simulink model "motor_speed_current_loop_model"  (R2023b)
settings: Solver=FixedStepDiscrete  StartTime=0.0  StopTime=simcfg.stop_time  FixedStep=simcfg.Ts_plant  RelTol=1e-3
values from neighbouring files (symbols this model uses):
  Kaw_id = 400.0    [motor_speed_current_loop_interface.sldd]
  Kaw_iq = 400.0    [motor_speed_current_loop_interface.sldd]
  Kaw_speed = 40.0    [motor_speed_current_loop_interface.sldd]
  Ki_id = 1072.4140625    [motor_speed_current_loop_interface.sldd]
  Ki_iq = 1072.4140625    [motor_speed_current_loop_interface.sldd]
  Ki_speed = 79.284461975097656    [motor_speed_current_loop_interface.sldd]
  Kp_id = 1.3320353031158447    [motor_speed_current_loop_interface.sldd]
  Kp_iq = 1.3320353031158447    [motor_speed_current_loop_interface.sldd]
  Kp_speed = 0.63092565536499023    [motor_speed_current_loop_interface.sldd]
  VLimitRatio = 0.57700002193450928    [motor_speed_current_loop_interface.sldd]
undefined symbols (not defined in the file or in its folder): current_pi_simcfg, inverter, motor, simcfg, speed_current_loop, speed_pi_simcfg
libraries: mcbplantlib x1, autolibpmsmexterior x1
settings Model: DataDictionary=motor_speed_current_loop_interface.sldd  Creator=user  LastModifiedBy=user
settings OptimizationCC: EnhancedBackFolding=on  PassReuseOutputArgsAs=Individual arguments  OptimizeBlockOrder=speed  DifferentSizesBufferReuse=on  OptimizationCustomize=off  EfficientTunableParamExpr=on
settings DebuggingCC: ParameterPrecisionLossMsg=none  ParameterTunabilityLossMsg=error
settings HardwareCC: ProdBitPerPointer=32  ProdBitPerSizeT=32  ProdBitPerPtrDiffT=32  ProdLargestAtomicInteger=Long  ProdLargestAtomicFloat=Double  ProdWordSize=32  ProdHWDeviceType=ARM Compatible->ARM Cortex  TargetLargestAtomicInteger=Long  TargetLargestAtomicFloat=Double  TargetIntDivRoundTo=Zero  TargetEndianess=LittleEndian  TargetHWDeviceType=ARM Compatible->ARM Cortex  ProdEqTarget=off
settings SFSimCC: MATLABDynamicMemAlloc=off
settings RTWCC: Description=Embedded Coder  SystemTargetFile=ert.tlc  GenCodeOnly=on  TemplateMakefile=ert_default_tmf  GenerateReport=on
settings CodeAppCC: ForceParamTrailComments=on  IgnoreCustomStorageClasses=off  OperatorAnnotations=on  SimulinkDataObjDesc=on  SFDataObjDesc=on  InsertBlockDesc=on
settings ERTTargetCC: TargetLangStandard=C99 (ISO)  CodeInterfacePackaging=Reusable function  ERTCustomFileTemplate=example_file_process.tlc

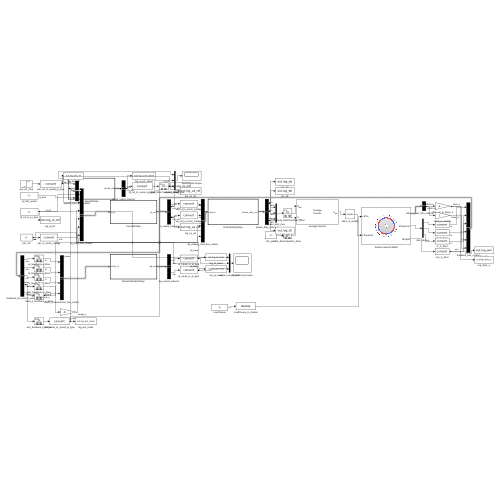
[thumbnail: Simulink's stored preview of the top-level diagram]
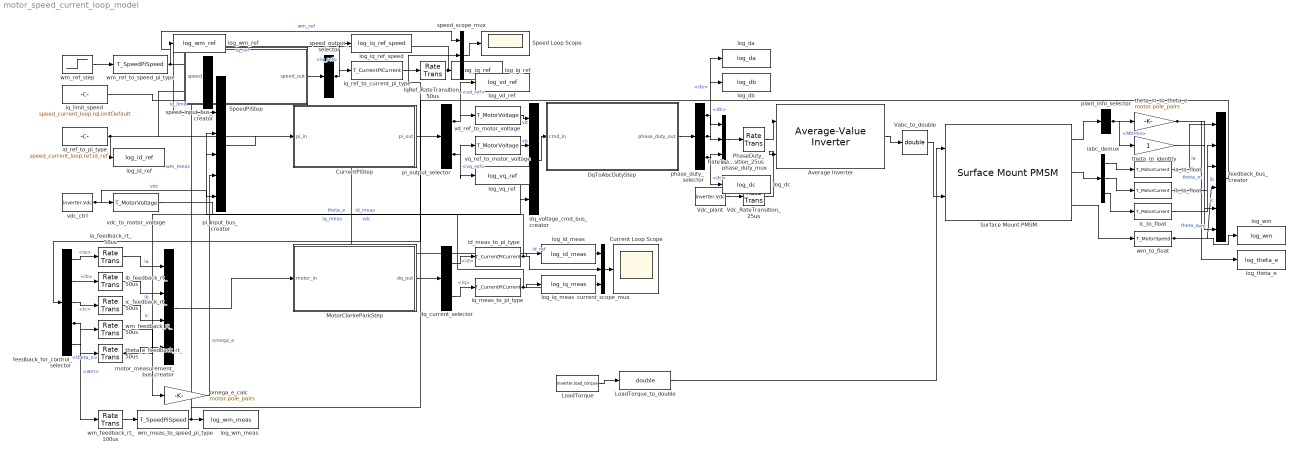
== system motor_speed_current_loop_model ==
  Average Inverter : mcbplantlib/Average-Value Inverter
  Current Loop Scope : Scope
  CurrentPiStep : Subsystem  TreatAsAtomicUnit=on  RTWFcnName=CurrentPiStep  RTWFileName=CurrentPiStep
      settings: RTWFcnNameOpts=User specified  RTWFileNameOpts=User specified
  DqToAbcDutyStep : Subsystem  TreatAsAtomicUnit=on  RTWFcnName=DqToAbcDutyStep  RTWFileName=DqToAbcDutyStep
      settings: RTWFcnNameOpts=User specified  RTWFileNameOpts=User specified
  IqRef_RateTransition_50us : RateTransition  OutPortSampleTime=simcfg.Ts_ctrl
  LoadTorque : Constant  Value=inverter.load_torque  OutDataTypeStr=T_MotorTorque  SampleTime=simcfg.Ts_plant
  LoadTorque_to_double : DataTypeConversion  OutDataTypeStr=double  SaturateOnIntegerOverflow=off  RndMeth=Floor
  MotorClarkeParkStep : Subsystem  TreatAsAtomicUnit=on  RTWFcnName=MotorClarkeParkStep  RTWFileName=MotorClarkeParkStep
      settings: RTWFcnNameOpts=User specified  RTWFileNameOpts=User specified
  PhaseDuty_RateTransition_25us : RateTransition  OutPortSampleTime=simcfg.Ts_plant
  Speed Loop Scope : Scope
  SpeedPiStep : Subsystem  TreatAsAtomicUnit=on  RTWFcnName=SpeedPiStep  RTWFileName=SpeedPiStep
      settings: RTWFcnNameOpts=User specified  RTWFileNameOpts=User specified
  Surface Mount PMSM : autolibpmsmexterior/Surface Mount PMSM  port_config=Torque  sim_type=Discrete  Ts=simcfg.Ts_plant  P=motor.pole_pairs  Rs=motor.Rs  Ldq_=motor.Ld  KConstText=Permanent flux linkage constant (lambda_pm):  lambda_pm=motor.psi_f  Ke=159.9771  Kt=1.323  mechanical=[motor.J, motor.B, 0]  idq0=[0 0]  theta_init=0  omega_init=0  KConst=motor.psi_f  lambda_pm_calc=motor.psi_f  RefBlkName='autolibpmsmexterior/Surface Mount PMSM'  aMode=5  Ldq="[0.0017      0.0017]"
  Vabc_to_double : DataTypeConversion  OutDataTypeStr=double  SaturateOnIntegerOverflow=off  RndMeth=Floor
  Vdc_RateTransition_25us : RateTransition  OutPortSampleTime=simcfg.Ts_plant
  Vdc_plant : Constant  Value=inverter.Vdc  OutDataTypeStr=T_MotorVoltage  SampleTime=simcfg.Ts_plant
  current_scope_mux : Mux  Inputs=3
  dq_current_selector : BusSelector  OutputSignals=id,iq
  dq_voltage_cmd_bus_creator : BusCreator  Inputs=4  OutDataTypeStr=Bus: open_loop_cmd_t  NonVirtualBus=on
  feedback_bus_creator : BusCreator  Inputs=6  OutDataTypeStr=Bus: plant_feedback_t  NonVirtualBus=on
  feedback_for_control_selector : BusSelector  OutputSignals=ia,ib,ic,wm,theta_e
  ia_feedback_rt_50us : RateTransition  OutPortSampleTime=simcfg.Ts_ctrl
  ia_to_float : DataTypeConversion  OutDataTypeStr=T_MotorCurrent  SaturateOnIntegerOverflow=off  RndMeth=Floor
  iabc_demux : Demux  Outputs=3
  ib_feedback_rt_50us : RateTransition  OutPortSampleTime=simcfg.Ts_ctrl
  ib_to_float : DataTypeConversion  OutDataTypeStr=T_MotorCurrent  SaturateOnIntegerOverflow=off  RndMeth=Floor
  ic_feedback_rt_50us : RateTransition  OutPortSampleTime=simcfg.Ts_ctrl
  ic_to_float : DataTypeConversion  OutDataTypeStr=T_MotorCurrent  SaturateOnIntegerOverflow=off  RndMeth=Floor
  id_meas_to_pi_type : DataTypeConversion  OutDataTypeStr=T_CurrentPiCurrent  SaturateOnIntegerOverflow=off  RndMeth=Floor
  id_ref_to_pi_type : Constant  Value=speed_current_loop.ref.id_ref  OutDataTypeStr=T_CurrentPiCurrent  SampleTime=simcfg.Ts_ctrl
  iq_limit_speed : Constant  Value=speed_current_loop.IqLimitDefault  OutDataTypeStr=T_SpeedPiCurrent  SampleTime=simcfg.Ts_speed
  iq_meas_to_pi_type : DataTypeConversion  OutDataTypeStr=T_CurrentPiCurrent  SaturateOnIntegerOverflow=off  RndMeth=Floor
  iq_ref_to_current_pi_type : DataTypeConversion  OutDataTypeStr=T_CurrentPiCurrent  SaturateOnIntegerOverflow=off  RndMeth=Floor
  log_da : ToWorkspace  VariableName=log_da  SaveFormat=Timeseries  SampleTime=-1
  log_db : ToWorkspace  VariableName=log_db  SaveFormat=Timeseries  SampleTime=-1
  log_dc : ToWorkspace  VariableName=log_dc  SaveFormat=Timeseries  SampleTime=-1
  log_id_meas : ToWorkspace  VariableName=log_id_meas  SaveFormat=Timeseries  SampleTime=-1
  log_id_ref : ToWorkspace  VariableName=log_id_ref  SaveFormat=Timeseries  SampleTime=-1
  log_iq_meas : ToWorkspace  VariableName=log_iq_meas  SaveFormat=Timeseries  SampleTime=-1
  log_iq_ref : ToWorkspace  VariableName=log_iq_ref  SaveFormat=Timeseries  SampleTime=-1
  log_iq_ref_speed : ToWorkspace  VariableName=log_iq_ref_speed  SaveFormat=Timeseries  SampleTime=-1
  log_theta_e : ToWorkspace  VariableName=log_theta_e  SaveFormat=Timeseries  SampleTime=-1
  log_vd_ref : ToWorkspace  VariableName=log_vd_ref  SaveFormat=Timeseries  SampleTime=-1
  log_vq_ref : ToWorkspace  VariableName=log_vq_ref  SaveFormat=Timeseries  SampleTime=-1
  log_wm : ToWorkspace  VariableName=log_wm  SaveFormat=Timeseries  SampleTime=-1
  log_wm_meas : ToWorkspace  VariableName=log_wm_meas  SaveFormat=Timeseries  SampleTime=-1
  log_wm_ref : ToWorkspace  VariableName=log_wm_ref  SaveFormat=Timeseries  SampleTime=-1
  motor_measurement_bus_creator : BusCreator  Inputs=4  OutDataTypeStr=Bus: motor_t  NonVirtualBus=on
  omega_e_calc : Gain  Gain=motor.pole_pairs  OutDataTypeStr=T_CurrentPiSpeed
  phase_duty_mux : Mux  Inputs=3
  phase_duty_selector : BusSelector  OutputSignals=da,db,dc
  pi_input_bus_creator : BusCreator  Inputs=6  OutDataTypeStr=Bus: current_pi_input_t  NonVirtualBus=on
  pi_output_selector : BusSelector  OutputSignals=vd_ref,vq_ref
  plant_info_selector : BusSelector  OutputSignals=MtrPos
  speed_input_bus_creator : BusCreator  Inputs=3  OutDataTypeStr=Bus: speed_pi_input_t  NonVirtualBus=on
  speed_output_selector : BusSelector  OutputSignals=iq_ref
  speed_scope_mux : Mux  Inputs=3
  theta_e_feedback_rt_50us : RateTransition  OutPortSampleTime=simcfg.Ts_ctrl
  theta_m_identity : Gain  OutDataTypeStr=T_MotorAngle
  theta_m_to_theta_e : Gain  Gain=motor.pole_pairs  OutDataTypeStr=T_MotorAngle
  vd_ref_to_motor_voltage : DataTypeConversion  OutDataTypeStr=T_MotorVoltage  SaturateOnIntegerOverflow=off  RndMeth=Floor
  vdc_ctrl : Constant  Value=inverter.Vdc  OutDataTypeStr=T_CurrentPiVoltage  SampleTime=simcfg.Ts_ctrl
  vdc_to_motor_voltage : DataTypeConversion  OutDataTypeStr=T_MotorVoltage  SaturateOnIntegerOverflow=off  RndMeth=Floor
  vq_ref_to_motor_voltage : DataTypeConversion  OutDataTypeStr=T_MotorVoltage  SaturateOnIntegerOverflow=off  RndMeth=Floor
  wm_feedback_rt_100us : RateTransition  OutPortSampleTime=simcfg.Ts_speed
  wm_feedback_rt_50us : RateTransition  OutPortSampleTime=simcfg.Ts_ctrl
  wm_meas_to_speed_pi_type : DataTypeConversion  OutDataTypeStr=T_SpeedPiSpeed  SaturateOnIntegerOverflow=off  RndMeth=Floor
  wm_ref_step : Step  Time=speed_current_loop.ref.wm_step_time  Before=speed_current_loop.ref.wm_before  After=speed_current_loop.ref.wm_after  SampleTime=simcfg.Ts_speed
  wm_ref_to_speed_pi_type : DataTypeConversion  OutDataTypeStr=T_SpeedPiSpeed  SaturateOnIntegerOverflow=off  RndMeth=Floor
  wm_to_float : DataTypeConversion  OutDataTypeStr=T_MotorSpeed  SaturateOnIntegerOverflow=off  RndMeth=Floor
  wires:
  wm_ref_step/1 -> wm_ref_to_speed_pi_type/1
  vdc_ctrl/1 -> vdc_to_motor_voltage/1, pi_input_bus_creator/6  "vdc"
  DqToAbcDutyStep/1(phase_duty_out) -> phase_duty_selector/1
  phase_duty_selector/1 -> phase_duty_mux/1, log_da/1  "<da>"
  phase_duty_selector/2 -> phase_duty_mux/2, log_db/1  "<db>"
  phase_duty_selector/3 -> phase_duty_mux/3, log_dc/1  "<dc>"
  phase_duty_mux/1 -> PhaseDuty_RateTransition_25us/1
  PhaseDuty_RateTransition_25us/1 -> Average Inverter/1
  Vdc_plant/1 -> Vdc_RateTransition_25us/1
  Vdc_RateTransition_25us/1 -> Average Inverter/2
  LoadTorque/1 -> LoadTorque_to_double/1
  LoadTorque_to_double/1 -> Surface Mount PMSM/1
  Average Inverter/1 -> Vabc_to_double/1
  Vabc_to_double/1 -> Surface Mount PMSM/2
  Surface Mount PMSM/1 -> plant_info_selector/1
  plant_info_selector/1 -> theta_m_to_theta_e/1, theta_m_identity/1  "<MtrPos>"
  Surface Mount PMSM/2 -> iabc_demux/1
  iabc_demux/1 -> ia_to_float/1
  iabc_demux/2 -> ib_to_float/1
  iabc_demux/3 -> ic_to_float/1
  Surface Mount PMSM/3 -> wm_to_float/1
  ia_to_float/1 -> feedback_bus_creator/1  "ia"
  ib_to_float/1 -> feedback_bus_creator/2  "ib"
  ic_to_float/1 -> feedback_bus_creator/3  "ic"
  wm_to_float/1 -> feedback_bus_creator/4, log_wm/1  "wm"
  theta_m_identity/1 -> feedback_bus_creator/5  "theta_m"
  theta_m_to_theta_e/1 -> feedback_bus_creator/6, log_theta_e/1  "theta_e"
  feedback_bus_creator/1 -> feedback_for_control_selector/1
  feedback_for_control_selector/1 -> ia_feedback_rt_50us/1  "<ia>"
  feedback_for_control_selector/2 -> ib_feedback_rt_50us/1  "<ib>"
  feedback_for_control_selector/3 -> ic_feedback_rt_50us/1  "<ic>"
  feedback_for_control_selector/4 -> wm_feedback_rt_50us/1, wm_feedback_rt_100us/1  "<wm>"
  feedback_for_control_selector/5 -> theta_e_feedback_rt_50us/1  "<theta_e>"
  ia_feedback_rt_50us/1 -> motor_measurement_bus_creator/1  "ia"
  ib_feedback_rt_50us/1 -> motor_measurement_bus_creator/2  "ib"
  ic_feedback_rt_50us/1 -> motor_measurement_bus_creator/3  "ic"
  theta_e_feedback_rt_50us/1 -> motor_measurement_bus_creator/4, dq_voltage_cmd_bus_creator/3  "theta_e"
  motor_measurement_bus_creator/1 -> MotorClarkeParkStep/1(motor_in)
  MotorClarkeParkStep/1(dq_out) -> dq_current_selector/1
  dq_current_selector/1 -> id_meas_to_pi_type/1  "<id>"
  dq_current_selector/2 -> iq_meas_to_pi_type/1  "<iq>"
  wm_feedback_rt_50us/1 -> omega_e_calc/1
  wm_ref_to_speed_pi_type/1 -> speed_input_bus_creator/1, log_wm_ref/1, speed_scope_mux/1  "wm_ref"
  wm_feedback_rt_100us/1 -> wm_meas_to_speed_pi_type/1
  wm_meas_to_speed_pi_type/1 -> speed_input_bus_creator/2, log_wm_meas/1, speed_scope_mux/2  "wm_meas"
  iq_limit_speed/1 -> speed_input_bus_creator/3  "iq_limit"
  speed_input_bus_creator/1 -> SpeedPiStep/1(speed_in)
  SpeedPiStep/1(speed_out) -> speed_output_selector/1
  speed_output_selector/1 -> iq_ref_to_current_pi_type/1, log_iq_ref_speed/1  "<iq_ref>"
  iq_ref_to_current_pi_type/1 -> IqRef_RateTransition_50us/1
  id_ref_to_pi_type/1 -> pi_input_bus_creator/1, log_id_ref/1, current_scope_mux/1  "id_ref"
  IqRef_RateTransition_50us/1 -> pi_input_bus_creator/2, log_iq_ref/1, speed_scope_mux/3  "iq_ref"
  id_meas_to_pi_type/1 -> pi_input_bus_creator/3, log_id_meas/1, current_scope_mux/2  "id_meas"
  iq_meas_to_pi_type/1 -> pi_input_bus_creator/4, log_iq_meas/1, current_scope_mux/3  "iq_meas"
  omega_e_calc/1 -> pi_input_bus_creator/5  "omega_e"
  CurrentPiStep/1(pi_out) -> pi_output_selector/1
  pi_output_selector/1 -> vd_ref_to_motor_voltage/1, log_vd_ref/1  "<vd_ref>"
  pi_output_selector/2 -> vq_ref_to_motor_voltage/1, log_vq_ref/1  "<vq_ref>"
  vd_ref_to_motor_voltage/1 -> dq_voltage_cmd_bus_creator/1  "vd"
  vq_ref_to_motor_voltage/1 -> dq_voltage_cmd_bus_creator/2  "vq"
  vdc_to_motor_voltage/1 -> dq_voltage_cmd_bus_creator/4  "vdc"
  pi_input_bus_creator/1 -> CurrentPiStep/1(pi_in)
  dq_voltage_cmd_bus_creator/1 -> DqToAbcDutyStep/1(cmd_in)
  current_scope_mux/1 -> Current Loop Scope/1
  speed_scope_mux/1 -> Speed Loop Scope/1

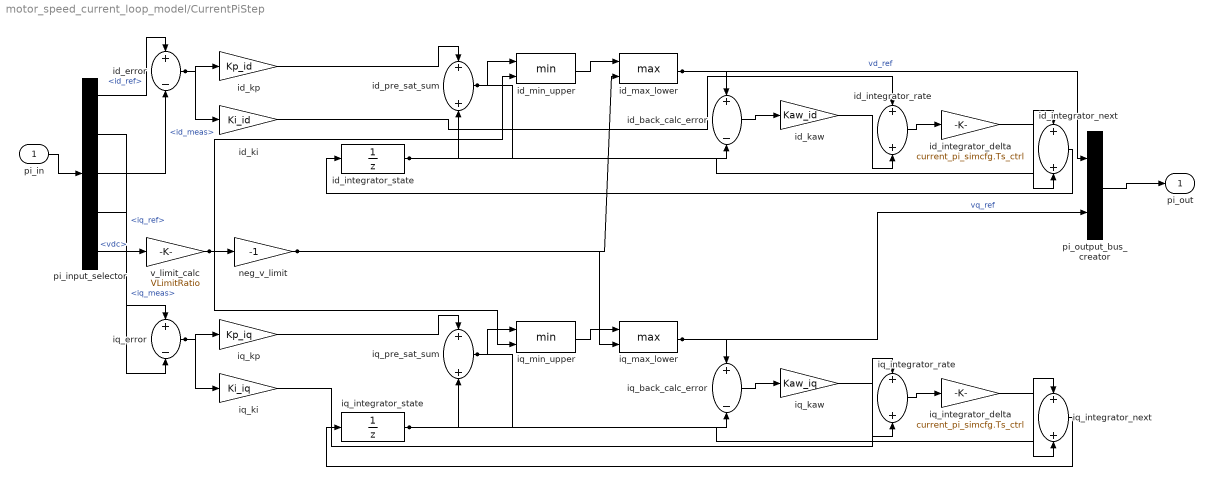
== system motor_speed_current_loop_model/CurrentPiStep ==
  pi_in : Inport  OutDataTypeStr=Bus: current_pi_input_t  BusOutputAsStruct=on
  id_back_calc_error : Sum  Inputs=+-  OutDataTypeStr=T_CurrentPiVoltage  AccumDataTypeStr=T_CurrentPiVoltage
  id_error : Sum  Inputs=+-  OutDataTypeStr=T_CurrentPiCurrent  AccumDataTypeStr=T_CurrentPiCurrent
  id_integrator_delta : Gain  Gain=current_pi_simcfg.Ts_ctrl  ParamDataTypeStr=T_CurrentPiFloat  OutDataTypeStr=T_CurrentPiVoltage
  id_integrator_next : Sum  OutDataTypeStr=T_CurrentPiVoltage  AccumDataTypeStr=T_CurrentPiVoltage
  id_integrator_rate : Sum  OutDataTypeStr=T_CurrentPiVoltage  AccumDataTypeStr=T_CurrentPiVoltage
  id_integrator_state : UnitDelay  SampleTime=current_pi_simcfg.Ts_ctrl  HasFrameUpgradeWarning=on
  id_kaw : Gain  Gain=Kaw_id  ParamDataTypeStr=T_CurrentPiGain  OutDataTypeStr=T_CurrentPiVoltage
  id_ki : Gain  Gain=Ki_id  ParamDataTypeStr=T_CurrentPiGain  OutDataTypeStr=T_CurrentPiVoltage
  id_kp : Gain  Gain=Kp_id  ParamDataTypeStr=T_CurrentPiGain  OutDataTypeStr=T_CurrentPiVoltage
  id_max_lower : MinMax  Function=max  Inputs=2
  id_min_upper : MinMax  Inputs=2
  id_pre_sat_sum : Sum  OutDataTypeStr=T_CurrentPiVoltage  AccumDataTypeStr=T_CurrentPiVoltage
  iq_back_calc_error : Sum  Inputs=+-  OutDataTypeStr=T_CurrentPiVoltage  AccumDataTypeStr=T_CurrentPiVoltage
  iq_error : Sum  Inputs=+-  OutDataTypeStr=T_CurrentPiCurrent  AccumDataTypeStr=T_CurrentPiCurrent
  iq_integrator_delta : Gain  Gain=current_pi_simcfg.Ts_ctrl  ParamDataTypeStr=T_CurrentPiFloat  OutDataTypeStr=T_CurrentPiVoltage
  iq_integrator_next : Sum  OutDataTypeStr=T_CurrentPiVoltage  AccumDataTypeStr=T_CurrentPiVoltage
  iq_integrator_rate : Sum  OutDataTypeStr=T_CurrentPiVoltage  AccumDataTypeStr=T_CurrentPiVoltage
  iq_integrator_state : UnitDelay  SampleTime=current_pi_simcfg.Ts_ctrl  HasFrameUpgradeWarning=on
  iq_kaw : Gain  Gain=Kaw_iq  ParamDataTypeStr=T_CurrentPiGain  OutDataTypeStr=T_CurrentPiVoltage
  iq_ki : Gain  Gain=Ki_iq  ParamDataTypeStr=T_CurrentPiGain  OutDataTypeStr=T_CurrentPiVoltage
  iq_kp : Gain  Gain=Kp_iq  ParamDataTypeStr=T_CurrentPiGain  OutDataTypeStr=T_CurrentPiVoltage
  iq_max_lower : MinMax  Function=max  Inputs=2
  iq_min_upper : MinMax  Inputs=2
  iq_pre_sat_sum : Sum  OutDataTypeStr=T_CurrentPiVoltage  AccumDataTypeStr=T_CurrentPiVoltage
  neg_v_limit : Gain  Gain=-1  ParamDataTypeStr=T_CurrentPiFloat  OutDataTypeStr=T_CurrentPiVoltage
  pi_input_selector : BusSelector  OutputSignals=id_ref,iq_ref,id_meas,iq_meas,vdc
  pi_output_bus_creator : BusCreator  Inputs=2  OutDataTypeStr=Bus: current_pi_output_t  NonVirtualBus=on
  v_limit_calc : Gain  Gain=VLimitRatio  ParamDataTypeStr=T_CurrentPiGain  OutDataTypeStr=T_CurrentPiVoltage
  pi_out : Outport  OutDataTypeStr=Bus: current_pi_output_t
  wires:
  pi_output_bus_creator/1 -> pi_out/1
  iq_integrator_next/1 -> iq_integrator_state/1
  iq_integrator_delta/1 -> iq_integrator_next/2
  iq_integrator_rate/1 -> iq_integrator_delta/1
  iq_kaw/1 -> iq_integrator_rate/2
  iq_ki/1 -> iq_integrator_rate/1
  iq_back_calc_error/1 -> iq_kaw/1
  iq_max_lower/1 -> pi_output_bus_creator/2, iq_back_calc_error/1  "vq_ref"
  iq_min_upper/1 -> iq_max_lower/1
  iq_pre_sat_sum/1 -> iq_back_calc_error/2, iq_min_upper/1
  iq_integrator_state/1 -> iq_integrator_next/1, iq_pre_sat_sum/2
  iq_kp/1 -> iq_pre_sat_sum/1
  iq_error/1 -> iq_ki/1, iq_kp/1
  pi_input_selector/4 -> iq_error/2  "<iq_meas>"
  pi_input_selector/2 -> iq_error/1  "<iq_ref>"
  id_integrator_next/1 -> id_integrator_state/1
  id_integrator_delta/1 -> id_integrator_next/2
  id_integrator_rate/1 -> id_integrator_delta/1
  id_kaw/1 -> id_integrator_rate/2
  id_ki/1 -> id_integrator_rate/1
  id_back_calc_error/1 -> id_kaw/1
  id_max_lower/1 -> pi_output_bus_creator/1, id_back_calc_error/1  "vd_ref"
  neg_v_limit/1 -> iq_max_lower/2, id_max_lower/2
  id_min_upper/1 -> id_max_lower/1
  id_pre_sat_sum/1 -> id_back_calc_error/2, id_min_upper/1
  id_integrator_state/1 -> id_integrator_next/1, id_pre_sat_sum/2
  id_kp/1 -> id_pre_sat_sum/1
  id_error/1 -> id_ki/1, id_kp/1
  pi_input_selector/3 -> id_error/2  "<id_meas>"
  pi_input_selector/1 -> id_error/1  "<id_ref>"
  v_limit_calc/1 -> iq_min_upper/2, id_min_upper/2, neg_v_limit/1
  pi_input_selector/5 -> v_limit_calc/1  "<vdc>"
  pi_in/1 -> pi_input_selector/1

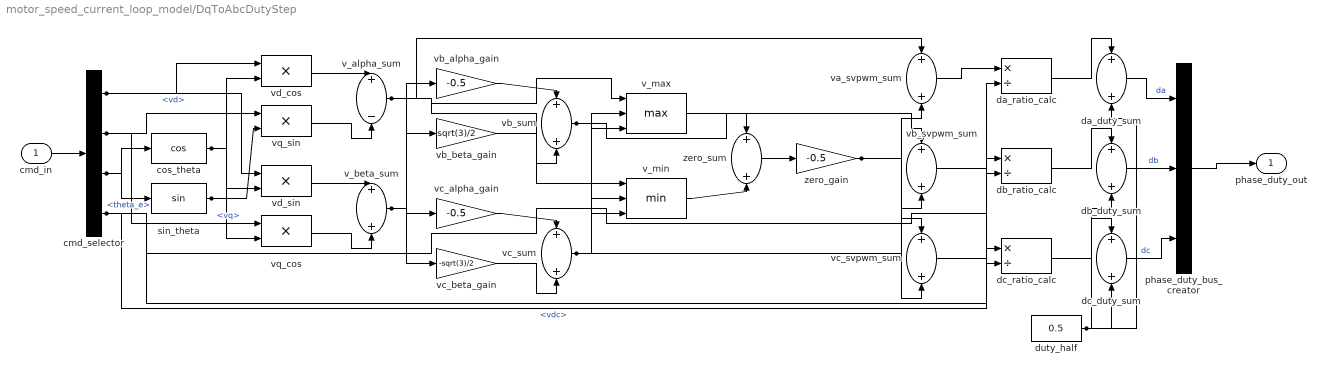
== system motor_speed_current_loop_model/DqToAbcDutyStep ==
  cmd_in : Inport  OutDataTypeStr=Bus: open_loop_cmd_t  BusOutputAsStruct=on
  cmd_selector : BusSelector  OutputSignals=vd,vq,theta_e,vdc
  cos_theta : Trigonometry  Operator=cos
  da_duty_sum : Sum  OutDataTypeStr=T_DutyRatio  AccumDataTypeStr=T_DutyRatio
  da_ratio_calc : Product  Inputs=*/  OutDataTypeStr=T_DutyRatio
  db_duty_sum : Sum  OutDataTypeStr=T_DutyRatio  AccumDataTypeStr=T_DutyRatio
  db_ratio_calc : Product  Inputs=*/  OutDataTypeStr=T_DutyRatio
  dc_duty_sum : Sum  OutDataTypeStr=T_DutyRatio  AccumDataTypeStr=T_DutyRatio
  dc_ratio_calc : Product  Inputs=*/  OutDataTypeStr=T_DutyRatio
  duty_half : Constant  Value=0.5  OutDataTypeStr=T_DutyRatio  SampleTime=simcfg.Ts_ctrl
  phase_duty_bus_creator : BusCreator  Inputs=3  OutDataTypeStr=Bus: phase_duty_t  NonVirtualBus=on
  sin_theta : Trigonometry
  v_alpha_sum : Sum  Inputs=+-  OutDataTypeStr=T_MotorVoltage  AccumDataTypeStr=T_MotorVoltage
  v_beta_sum : Sum  OutDataTypeStr=T_MotorVoltage  AccumDataTypeStr=T_MotorVoltage
  v_max : MinMax  Function=max  Inputs=3
  v_min : MinMax  Inputs=3
  va_svpwm_sum : Sum  OutDataTypeStr=T_MotorVoltage  AccumDataTypeStr=T_MotorVoltage
  vb_alpha_gain : Gain  Gain=-0.5  ParamDataTypeStr=T_MotorFloat  OutDataTypeStr=T_MotorVoltage
  vb_beta_gain : Gain  Gain=sqrt(3)/2  ParamDataTypeStr=T_MotorFloat  OutDataTypeStr=T_MotorVoltage
  vb_sum : Sum  OutDataTypeStr=T_MotorVoltage  AccumDataTypeStr=T_MotorVoltage
  vb_svpwm_sum : Sum  OutDataTypeStr=T_MotorVoltage  AccumDataTypeStr=T_MotorVoltage
  vc_alpha_gain : Gain  Gain=-0.5  ParamDataTypeStr=T_MotorFloat  OutDataTypeStr=T_MotorVoltage
  vc_beta_gain : Gain  Gain=-sqrt(3)/2  ParamDataTypeStr=T_MotorFloat  OutDataTypeStr=T_MotorVoltage
  vc_sum : Sum  OutDataTypeStr=T_MotorVoltage  AccumDataTypeStr=T_MotorVoltage
  vc_svpwm_sum : Sum  OutDataTypeStr=T_MotorVoltage  AccumDataTypeStr=T_MotorVoltage
  vd_cos : Product  Inputs=**  OutDataTypeStr=T_MotorVoltage
  vd_sin : Product  Inputs=**  OutDataTypeStr=T_MotorVoltage
  vq_cos : Product  Inputs=**  OutDataTypeStr=T_MotorVoltage
  vq_sin : Product  Inputs=**  OutDataTypeStr=T_MotorVoltage
  zero_gain : Gain  Gain=-0.5  ParamDataTypeStr=T_MotorFloat  OutDataTypeStr=T_MotorVoltage
  zero_sum : Sum  OutDataTypeStr=T_MotorVoltage  AccumDataTypeStr=T_MotorVoltage
  phase_duty_out : Outport  OutDataTypeStr=Bus: phase_duty_t
  wires:
  phase_duty_bus_creator/1 -> phase_duty_out/1
  dc_duty_sum/1 -> phase_duty_bus_creator/3  "dc"
  db_duty_sum/1 -> phase_duty_bus_creator/2  "db"
  da_duty_sum/1 -> phase_duty_bus_creator/1  "da"
  duty_half/1 -> dc_duty_sum/2, db_duty_sum/2, da_duty_sum/2
  dc_ratio_calc/1 -> dc_duty_sum/1
  db_ratio_calc/1 -> db_duty_sum/1
  da_ratio_calc/1 -> da_duty_sum/1
  vc_svpwm_sum/1 -> dc_ratio_calc/1
  vb_svpwm_sum/1 -> db_ratio_calc/1
  cmd_selector/4 -> dc_ratio_calc/2, db_ratio_calc/2, da_ratio_calc/2  "<vdc>"
  va_svpwm_sum/1 -> da_ratio_calc/1
  zero_gain/1 -> vc_svpwm_sum/2, vb_svpwm_sum/2, va_svpwm_sum/2
  zero_sum/1 -> zero_gain/1
  v_min/1 -> zero_sum/2
  v_max/1 -> zero_sum/1
  vc_sum/1 -> vc_svpwm_sum/1, v_min/3, v_max/3
  vb_sum/1 -> vb_svpwm_sum/1, v_min/2, v_max/2
  vc_beta_gain/1 -> vc_sum/2
  vc_alpha_gain/1 -> vc_sum/1
  vb_beta_gain/1 -> vb_sum/2
  vb_alpha_gain/1 -> vb_sum/1
  v_beta_sum/1 -> vc_beta_gain/1, vb_beta_gain/1
  v_alpha_sum/1 -> va_svpwm_sum/1, v_min/1, v_max/1, vc_alpha_gain/1, vb_alpha_gain/1
  vq_cos/1 -> v_beta_sum/2
  vd_sin/1 -> v_beta_sum/1
  vq_sin/1 -> v_alpha_sum/2
  vd_cos/1 -> v_alpha_sum/1
  sin_theta/1 -> vd_sin/2, vq_sin/2
  cmd_selector/2 -> vq_cos/1, vq_sin/1  "<vq>"
  cos_theta/1 -> vq_cos/2, vd_cos/2
  cmd_selector/1 -> vd_sin/1, vd_cos/1  "<vd>"
  cmd_selector/3 -> sin_theta/1, cos_theta/1  "<theta_e>"
  cmd_in/1 -> cmd_selector/1

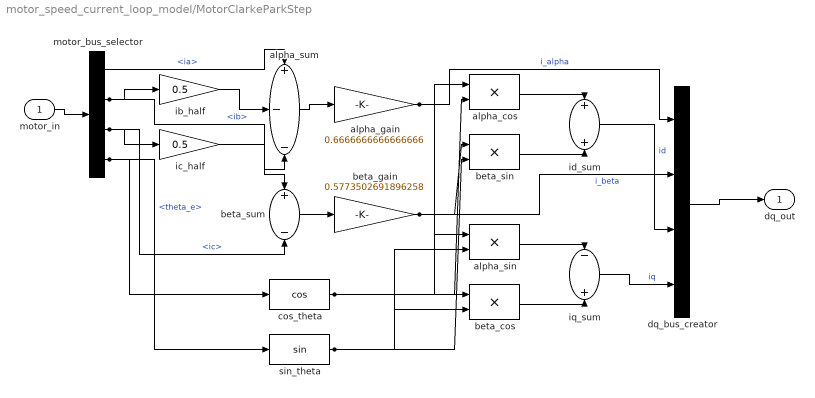
== system motor_speed_current_loop_model/MotorClarkeParkStep ==
  motor_in : Inport  OutDataTypeStr=Bus: motor_t  BusOutputAsStruct=on
  alpha_cos : Product  Inputs=**  OutDataTypeStr=T_MotorCurrent  SaturateOnIntegerOverflow=on
  alpha_gain : Gain  Gain=0.6666666666666666  ParamDataTypeStr=T_MotorCurrent  OutDataTypeStr=T_MotorCurrent  SaturateOnIntegerOverflow=on
  alpha_sin : Product  Inputs=**  OutDataTypeStr=T_MotorCurrent  SaturateOnIntegerOverflow=on
  alpha_sum : Sum  Inputs=+--  OutDataTypeStr=T_MotorCurrent  AccumDataTypeStr=T_MotorCurrent  SaturateOnIntegerOverflow=on
  beta_cos : Product  Inputs=**  OutDataTypeStr=T_MotorCurrent  SaturateOnIntegerOverflow=on
  beta_gain : Gain  Gain=0.5773502691896258  ParamDataTypeStr=T_MotorCurrent  OutDataTypeStr=T_MotorCurrent  SaturateOnIntegerOverflow=on
  beta_sin : Product  Inputs=**  OutDataTypeStr=T_MotorCurrent  SaturateOnIntegerOverflow=on
  beta_sum : Sum  Inputs=+-  OutDataTypeStr=T_MotorCurrent  AccumDataTypeStr=T_MotorCurrent  SaturateOnIntegerOverflow=on
  cos_theta : Trigonometry  Operator=cos
  dq_bus_creator : BusCreator  Inputs=4  OutDataTypeStr=Bus: motor_dq_t  NonVirtualBus=on
  ib_half : Gain  Gain=0.5  ParamDataTypeStr=T_MotorCurrent  OutDataTypeStr=T_MotorCurrent  SaturateOnIntegerOverflow=on
  ic_half : Gain  Gain=0.5  ParamDataTypeStr=T_MotorCurrent  OutDataTypeStr=T_MotorCurrent  SaturateOnIntegerOverflow=on
  id_sum : Sum  OutDataTypeStr=T_MotorCurrent  AccumDataTypeStr=T_MotorCurrent  SaturateOnIntegerOverflow=on
  iq_sum : Sum  Inputs=-+  OutDataTypeStr=T_MotorCurrent  AccumDataTypeStr=T_MotorCurrent  SaturateOnIntegerOverflow=on
  motor_bus_selector : BusSelector  OutputSignals=ia,ib,ic,theta_e
  sin_theta : Trigonometry
  dq_out : Outport  OutDataTypeStr=Bus: motor_dq_t
  wires:
  dq_bus_creator/1 -> dq_out/1
  iq_sum/1 -> dq_bus_creator/4  "iq"
  id_sum/1 -> dq_bus_creator/3  "id"
  beta_cos/1 -> iq_sum/2
  alpha_sin/1 -> iq_sum/1
  beta_sin/1 -> id_sum/2
  alpha_cos/1 -> id_sum/1
  sin_theta/1 -> alpha_sin/2, beta_sin/2
  beta_gain/1 -> dq_bus_creator/2, beta_cos/1, beta_sin/1  "i_beta"
  cos_theta/1 -> beta_cos/2, alpha_cos/2
  alpha_gain/1 -> dq_bus_creator/1, alpha_sin/1, alpha_cos/1  "i_alpha"
  motor_bus_selector/4 -> sin_theta/1, cos_theta/1  "<theta_e>"
  beta_sum/1 -> beta_gain/1
  alpha_sum/1 -> alpha_gain/1
  ic_half/1 -> alpha_sum/3
  ib_half/1 -> alpha_sum/2
  motor_bus_selector/3 -> beta_sum/2, ic_half/1  "<ic>"
  motor_bus_selector/2 -> beta_sum/1, ib_half/1  "<ib>"
  motor_bus_selector/1 -> alpha_sum/1  "<ia>"
  motor_in/1 -> motor_bus_selector/1

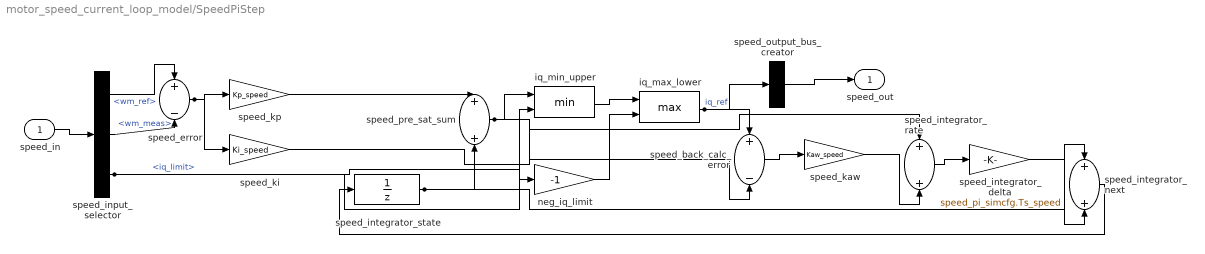
== system motor_speed_current_loop_model/SpeedPiStep ==
  speed_in : Inport  OutDataTypeStr=Bus: speed_pi_input_t  BusOutputAsStruct=on
  iq_max_lower : MinMax  Function=max  Inputs=2
  iq_min_upper : MinMax  Inputs=2
  neg_iq_limit : Gain  Gain=-1  ParamDataTypeStr=T_SpeedPiFloat  OutDataTypeStr=T_SpeedPiCurrent
  speed_back_calc_error : Sum  Inputs=+-  OutDataTypeStr=T_SpeedPiCurrent  AccumDataTypeStr=T_SpeedPiCurrent
  speed_error : Sum  Inputs=+-  OutDataTypeStr=T_SpeedPiSpeed  AccumDataTypeStr=T_SpeedPiSpeed
  speed_input_selector : BusSelector  OutputSignals=wm_ref,wm_meas,iq_limit
  speed_integrator_delta : Gain  Gain=speed_pi_simcfg.Ts_speed  ParamDataTypeStr=T_SpeedPiFloat  OutDataTypeStr=T_SpeedPiCurrent
  speed_integrator_next : Sum  OutDataTypeStr=T_SpeedPiCurrent  AccumDataTypeStr=T_SpeedPiCurrent
  speed_integrator_rate : Sum  OutDataTypeStr=T_SpeedPiCurrent  AccumDataTypeStr=T_SpeedPiCurrent
  speed_integrator_state : UnitDelay  SampleTime=speed_pi_simcfg.Ts_speed  HasFrameUpgradeWarning=on
  speed_kaw : Gain  Gain=Kaw_speed  ParamDataTypeStr=T_SpeedPiGain  OutDataTypeStr=T_SpeedPiCurrent
  speed_ki : Gain  Gain=Ki_speed  ParamDataTypeStr=T_SpeedPiGain  OutDataTypeStr=T_SpeedPiCurrent
  speed_kp : Gain  Gain=Kp_speed  ParamDataTypeStr=T_SpeedPiGain  OutDataTypeStr=T_SpeedPiCurrent
  speed_output_bus_creator : BusCreator  Inputs=1  OutDataTypeStr=Bus: speed_pi_output_t  NonVirtualBus=on
  speed_pre_sat_sum : Sum  OutDataTypeStr=T_SpeedPiCurrent  AccumDataTypeStr=T_SpeedPiCurrent
  speed_out : Outport  OutDataTypeStr=Bus: speed_pi_output_t
  wires:
  speed_integrator_next/1 -> speed_integrator_state/1
  speed_integrator_delta/1 -> speed_integrator_next/2
  speed_integrator_rate/1 -> speed_integrator_delta/1
  speed_kaw/1 -> speed_integrator_rate/2
  speed_ki/1 -> speed_integrator_rate/1
  speed_back_calc_error/1 -> speed_kaw/1
  speed_output_bus_creator/1 -> speed_out/1
  iq_max_lower/1 -> speed_back_calc_error/1, speed_output_bus_creator/1  "iq_ref"
  neg_iq_limit/1 -> iq_max_lower/2
  iq_min_upper/1 -> iq_max_lower/1
  speed_input_selector/3 -> neg_iq_limit/1, iq_min_upper/2  "<iq_limit>"
  speed_pre_sat_sum/1 -> speed_back_calc_error/2, iq_min_upper/1
  speed_integrator_state/1 -> speed_integrator_next/1, speed_pre_sat_sum/2
  speed_kp/1 -> speed_pre_sat_sum/1
  speed_error/1 -> speed_ki/1, speed_kp/1
  speed_input_selector/2 -> speed_error/2  "<wm_meas>"
  speed_input_selector/1 -> speed_error/1  "<wm_ref>"
  speed_in/1 -> speed_input_selector/1
